simulink model "model7_9"  (R2024b)
settings: Solver=VariableStepAuto  StartTime=0.0  StopTime=10.0  RelTol=1e-3
settings Model: Creator=Xist  LastModifiedBy=Xist

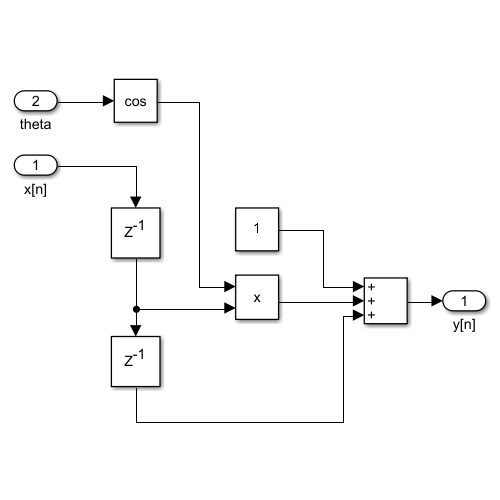
[thumbnail: Simulink's stored preview of the top-level diagram]
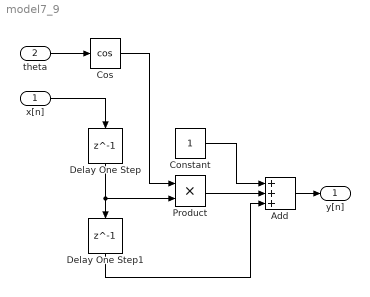
== system model7_9 ==
  x[n] : Inport
  theta : Inport  Port=2
  Add : Sum  Inputs=+++
  Constant : Constant
  Cos : Trigonometry  Operator=cos
  Delay One Step : Delay  DelayLength=1
  Delay One Step1 : Delay  DelayLength=1
  Product : Product
  y[n] : Outport
  wires:
  Delay One Step/1 -> Product/2, Delay One Step1/1
  Add/1 -> y[n]/1
  x[n]/1 -> Delay One Step/1
  Delay One Step1/1 -> Add/3
  Product/1 -> Add/2
  Constant/1 -> Add/1
  theta/1 -> Cos/1
  Cos/1 -> Product/1
